simulink model "Follower_Agent"  (R2014b)
settings: Solver=ode3  SolverMode=SingleTasking  StartTime=0.0  StopTime=10.0  FixedStep=sampleTimes.main  RelTol=1e-3
model workspace (MAT data in the model file):
  vehicle = 0
undefined symbols (not defined in the file or in its folder): delays, sampleTimes
libraries: simulink x18
(part 1 of 2)
settings Model: ParameterArgumentNames=vehicle  Creator=uos  LastModifiedBy=uos

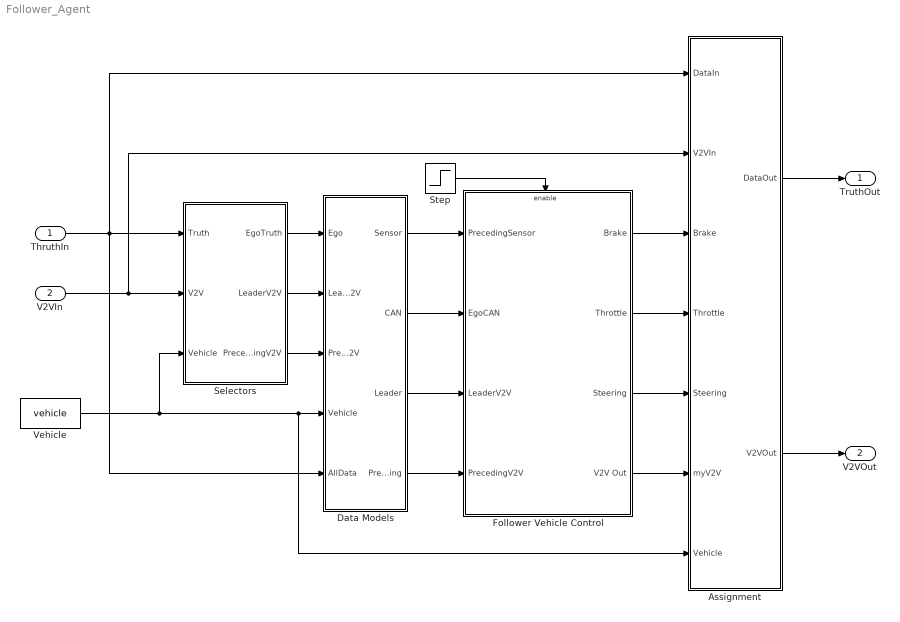
== system Follower_Agent ==
  ThruthIn : Inport  OutDataTypeStr=Bus: VehicleBus  PortDimensions=10  BusOutputAsStruct=on
  V2VIn : Inport  Port=2  OutDataTypeStr=Bus: V2VBus  PortDimensions=10  SampleTime=0  BusOutputAsStruct=on
  Assignment : Subsystem
  Data Models : Subsystem
  Follower Vehicle Control : Subsystem
  Selectors : Subsystem
  Step : Step  Time=vehicle*2  SampleTime=0
  Vehicle : Constant  Value=vehicle  OutDataTypeStr=int32
  TruthOut : Outport  OutDataTypeStr=Bus: VehicleBus  PortDimensions=10  BusOutputAsStruct=on
  V2VOut : Outport  Port=2  OutDataTypeStr=Bus: V2VBus  PortDimensions=10  BusOutputAsStruct=on
  wires:
  ThruthIn/1 -> Data Models/5(AllData), Assignment/1(DataIn), Selectors/1(Truth)
  Assignment/1(DataOut) -> TruthOut/1
  Vehicle/1 -> Data Models/4(Vehicle), Assignment/7(Vehicle), Selectors/3(Vehicle)
  Follower Vehicle Control/1(Brake) -> Assignment/3(Brake)
  Follower Vehicle Control/2(Throttle) -> Assignment/4(Throttle)
  Follower Vehicle Control/3(Steering) -> Assignment/5(Steering)
  V2VIn/1 -> Assignment/2(V2VIn), Selectors/2(V2V)
  Assignment/2(V2VOut) -> V2VOut/1
  Follower Vehicle Control/4(V2V Out) -> Assignment/6(myV2V)
  Selectors/1(EgoTruth) -> Data Models/1(Ego)
  Selectors/2(LeaderV2V) -> Data Models/2(LeaderV2V)
  Selectors/3(PrecedingV2V) -> Data Models/3(PrecedingV2V)
  Data Models/1(Sensor) -> Follower Vehicle Control/1(PrecedingSensor)
  Data Models/2(CAN) -> Follower Vehicle Control/2(EgoCAN)
  Data Models/3(Leader) -> Follower Vehicle Control/3(LeaderV2V)
  Data Models/4(Preceding) -> Follower Vehicle Control/4(PrecedingV2V)
  Step/1 -> Follower Vehicle Control/Enable

== system Follower_Agent/Assignment ==
  DataIn : Inport
  V2VIn : Inport  Port=2
  Brake : Inport  Port=3
  Throttle : Inport  Port=4
  Steering : Inport  Port=5
  myV2V : Inport  Port=6
  Vehicle : Inport  Port=7
  Clutch pedal value : Constant  Value=0
  Gear : Constant  Value=5  OutDataTypeStr=int32
  MATLAB Function : MATLAB Function  TreatAsAtomicUnit=on
  DataOut : Outport
  V2VOut : Outport  Port=2
  wires:
  Vehicle/1 -> MATLAB Function/9(vehicle)
  DataIn/1 -> MATLAB Function/1(dataIn)
  Brake/1 -> MATLAB Function/4(brake)
  MATLAB Function/1(dataOut) -> DataOut/1
  Throttle/1 -> MATLAB Function/5(throttle)
  Steering/1 -> MATLAB Function/8(steering)
  V2VIn/1 -> MATLAB Function/2(V2Vin)
  myV2V/1 -> MATLAB Function/3(myV2V)
  MATLAB Function/2(V2Vout) -> V2VOut/1
  Gear/1 -> MATLAB Function/6(gear)
  Clutch pedal value/1 -> MATLAB Function/7(clutch)

== system Follower_Agent/Data Models ==
  Ego : Inport
  LeaderV2V : Inport  Port=2
  PrecedingV2V : Inport  Port=3
  Vehicle : Inport  Port=4
  AllData : Inport  Port=5
  CAN Model : Subsystem
  Comms Model : Subsystem
  Sensor Model1 : Subsystem
  Sensor : Outport
  CAN : Outport  Port=2
  Leader : Outport  Port=3
  Preceding : Outport  Port=4
  wires:
  CAN Model/1(EgoCAN) -> CAN/1
  LeaderV2V/1 -> Comms Model/1(LeaderV2VIn)
  PrecedingV2V/1 -> Comms Model/2(PrecedingV2VIn)
  Comms Model/1(LeaderV2V) -> Leader/1
  Comms Model/2(PrecedingV2V) -> Preceding/1
  Vehicle/1 -> CAN Model/2(Vehicle), Sensor Model1/2(Vehicle)
  Ego/1 -> Sensor Model1/3(Ego), CAN Model/1(EgoData)
  AllData/1 -> Sensor Model1/1(AllData)
  Sensor Model1/1(Radar Data) -> Sensor/1

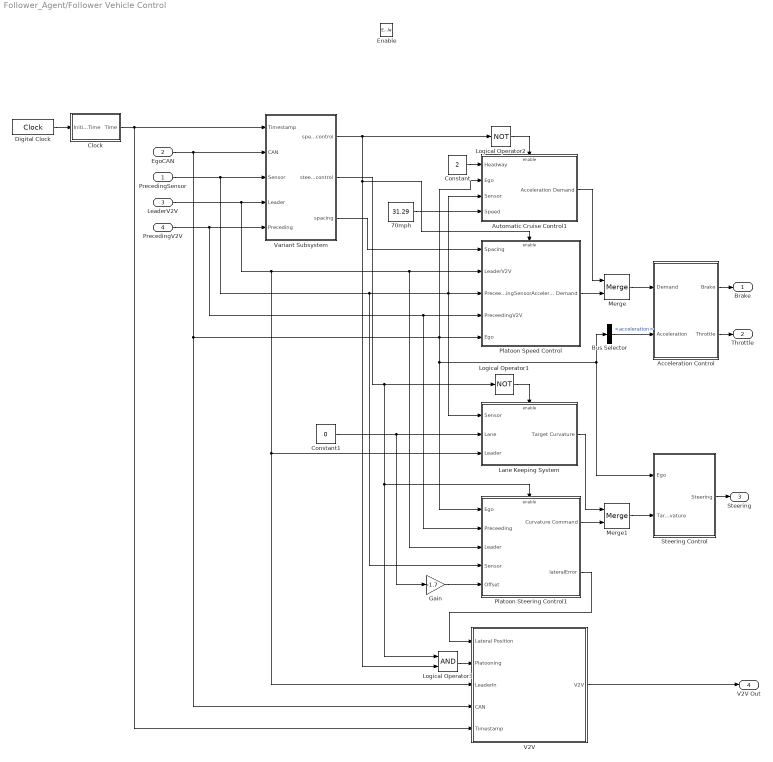
== system Follower_Agent/Follower Vehicle Control ==
  PrecedingSensor : Inport
  EgoCAN : Inport  Port=2
  LeaderV2V : Inport  Port=3
  PrecedingV2V : Inport  Port=4
  Enable : EnablePort
  70mph : Constant  Value=31.29
  Acceleration Control : Subsystem
  Automatic Cruise Control1 : Subsystem
  Bus Selector : BusSelector  OutputSignals=acceleration
  Clock : Subsystem
  Constant : Constant  Value=2
  Constant1 : Constant  Value=0
  Digital Clock : DigitalClock  SampleTime=sampleTimes.control
  Gain : Gain  Gain=-1.7
  Lane Keeping System : Subsystem
  Logical Operator1 : Logic  Operator=NOT  AllPortsSameDT=off  OutDataTypeStr=boolean
  Logical Operator2 : Logic  Operator=NOT  AllPortsSameDT=off  OutDataTypeStr=boolean
  Logical Operator3 : Logic  AllPortsSameDT=off  OutDataTypeStr=boolean
  Merge : Merge
  Merge1 : Merge
  Platoon Speed Control : Subsystem
  Platoon Steering Control1 : Subsystem
  Steering Control : Subsystem
  V2V : Subsystem
  Variant Subsystem : Subsystem  Variant=on  OverrideUsingVariant=Variant
  Brake : Outport
  Throttle : Outport  Port=2
  Steering : Outport  Port=3
  V2V Out : Outport  Port=4
  wires:
  Bus Selector/1 -> Acceleration Control/2(Acceleration)  "<acceleration>"
  Acceleration Control/1(Brake) -> Brake/1
  Acceleration Control/2(Throttle) -> Throttle/1
  Steering Control/1(Steering) -> Steering/1
  LeaderV2V/1 -> Variant Subsystem/4(Leader), Lane Keeping System/3(Leader), V2V/3(LeaderIn), Platoon Steering Control1/3(Leader), Platoon Speed Control/2(LeaderV2V)
  PrecedingSensor/1 -> Variant Subsystem/3(Sensor), Platoon Steering Control1/4(Sensor), Automatic Cruise Control1/3(Sensor), Lane Keeping System/1(Sensor), Platoon Speed Control/3(PreceedingSensor)
  Merge/1 -> Acceleration Control/1(Demand)
  Variant Subsystem/1(speed_control) -> Logical Operator3/2, Platoon Speed Control/Enable, Logical Operator2/1
  Merge1/1 -> Steering Control/2(Target Curvature)
  V2V/1(V2V) -> V2V Out/1
  PrecedingV2V/1 -> Variant Subsystem/5(Preceding), Platoon Steering Control1/2(Preceeding), Platoon Speed Control/4(PreceedingV2V)
  Digital Clock/1 -> Clock/1(Initial Time)
  Clock/1(Time) -> Variant Subsystem/1(Timestamp), V2V/5(Timestamp)
  Logical Operator2/1 -> Automatic Cruise Control1/Enable
  Constant/1 -> Automatic Cruise Control1/1(Headway)
  Variant Subsystem/3(spacing) -> Platoon Speed Control/1(Spacing)
  Automatic Cruise Control1/1(Acceleration Demand) -> Merge/1
  Platoon Speed Control/1(Acceleration Demand) -> Merge/2
  Logical Operator1/1 -> Lane Keeping System/Enable
  Variant Subsystem/2(steering_control) -> Logical Operator1/1, Platoon Steering Control1/Enable, Logical Operator3/1
  EgoCAN/1 -> Variant Subsystem/2(CAN), Automatic Cruise Control1/2(Ego), Platoon Steering Control1/1(Ego), Steering Control/1(Ego), Bus Selector/1, Platoon Speed Control/5(Ego), V2V/4(CAN)
  Lane Keeping System/1(Target Curvature) -> Merge1/1
  Platoon Steering Control1/1(Curvature Command) -> Merge1/2
  Platoon Steering Control1/2(lateralError) -> V2V/1(Lateral Position)
  Logical Operator3/1 -> V2V/2(Platooning)
  Constant1/1 -> Gain/1, Lane Keeping System/2(Lane)
  Gain/1 -> Platoon Steering Control1/5(Offset)
  70mph/1 -> Automatic Cruise Control1/4(Speed)

== system Follower_Agent/Selectors ==
  Truth : Inport
  V2V : Inport  Port=2
  Vehicle : Inport  Port=3
  MATLAB Function : MATLAB Function  TreatAsAtomicUnit=on
  EgoTruth : Outport
  LeaderV2V : Outport  Port=2
  PrecedingV2V : Outport  Port=3
  wires:
  Truth/1 -> MATLAB Function/1(data)
  Vehicle/1 -> MATLAB Function/3(vehicle)
  MATLAB Function/1(egoTruth) -> EgoTruth/1
  V2V/1 -> MATLAB Function/2(V2V)
  MATLAB Function/2(leaderV2V) -> LeaderV2V/1
  MATLAB Function/3(precedingV2V) -> PrecedingV2V/1

== system Follower_Agent/Data Models/CAN Model ==
  EgoData : Inport
  Vehicle : Inport  Port=2
  CAN Model : Subsystem
  EgoCAN : Outport
  wires:
  EgoData/1 -> CAN Model/1(Data)
  CAN Model/1(CAN) -> EgoCAN/1
  Vehicle/1 -> CAN Model/2(Vehicle)

== system Follower_Agent/Data Models/Comms Model ==
  LeaderV2VIn : Inport
  PrecedingV2VIn : Inport  Port=2
  Comms Delay : Subsystem
  Comms Delay1 : Subsystem
  Constant : Constant  Value=0
  Constant1 : Constant  Value=0
  LeaderV2V : Outport
  PrecedingV2V : Outport  Port=2
  wires:
  LeaderV2VIn/1 -> Comms Delay/1(Data)
  Comms Delay/1(V2V) -> LeaderV2V/1
  PrecedingV2VIn/1 -> Comms Delay1/1(Data)
  Comms Delay1/1(V2V) -> PrecedingV2V/1
  Constant/1 -> Comms Delay1/2(Delay)
  Constant1/1 -> Comms Delay/2(Delay)

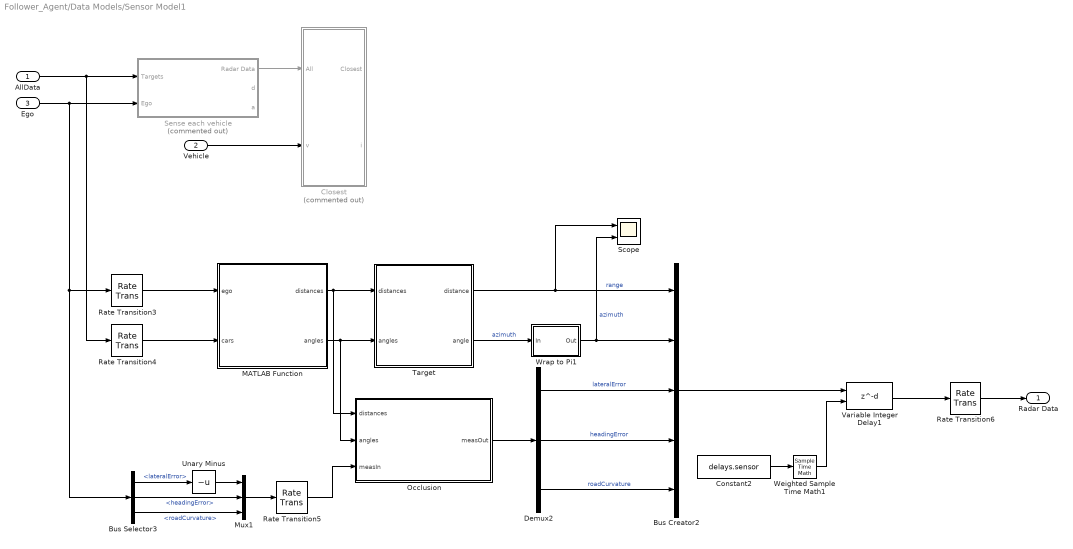
== system Follower_Agent/Data Models/Sensor Model1 ==
  AllData : Inport
  Vehicle : Inport  Port=2
  Ego : Inport  Port=3
  Bus Creator2 : BusCreator  Inputs=5  OutDataTypeStr=Bus: SensorData  NonVirtualBus=on
  Bus Selector3 : BusSelector  OutputSignals=data.lateralError,data.headingError,data.roadCurvature
  Closest : MATLAB Function  Commented=on  TreatAsAtomicUnit=on
  Constant2 : Constant  Value=delays.sensor
  Demux2 : Demux  Outputs=3
  MATLAB Function : MATLAB Function  TreatAsAtomicUnit=on
  Mux1 : Mux  Inputs=3
  Occlusion : MATLAB Function  TreatAsAtomicUnit=on
  Rate Transition3 : RateTransition  OutPortSampleTime=sampleTimes.main
  Rate Transition4 : RateTransition  OutPortSampleTime=sampleTimes.main
  Rate Transition5 : RateTransition  OutPortSampleTime=sampleTimes.main
  Rate Transition6 : RateTransition  OutPortSampleTime=sampleTimes.sensor
  Scope : Scope  NumInputPorts=2
      settings: TimeRange=23.7  YMin=0~-0.5  YMax=100~0
  Sense each vehicle : Subsystem  Commented=on  TreatAsAtomicUnit=on
  Target : MATLAB Function  TreatAsAtomicUnit=on
  Unary Minus : UnaryMinus
  Variable Integer Delay1 : Delay  DelayLengthSource=Input port
      settings: InputPortMap=u0,p1
  Weighted Sample Time Math1 : SampleTimeMath  TsampMathOp=/
  Wrap to Pi1 : Subsystem
  Radar Data : Outport
  wires:
  Vehicle/1 -> Closest/2(v)
  AllData/1 -> Rate Transition4/1, Sense each vehicle/1(Targets)
  Ego/1 -> Bus Selector3/1, Rate Transition3/1, Sense each vehicle/2(Ego)
  Sense each vehicle/1(Radar Data) -> Closest/1(All)
  Rate Transition3/1 -> MATLAB Function/1(ego)
  Rate Transition4/1 -> MATLAB Function/2(cars)
  MATLAB Function/1(distances) -> Occlusion/1(distances), Target/1(distances)
  MATLAB Function/2(angles) -> Occlusion/2(angles), Target/2(angles)
  Demux2/1 -> Bus Creator2/3  "lateralError"
  Demux2/2 -> Bus Creator2/4  "headingError"
  Demux2/3 -> Bus Creator2/5  "roadCurvature"
  Target/2(angle) -> Wrap to Pi1/1(In)  "azimuth"
  Target/1(distance) -> Scope/1, Bus Creator2/1  "range"
  Mux1/1 -> Rate Transition5/1
  Bus Selector3/1 -> Unary Minus/1  "<lateralError>"
  Bus Selector3/2 -> Mux1/2  "<headingError>"
  Bus Selector3/3 -> Mux1/3  "<roadCurvature>"
  Rate Transition5/1 -> Occlusion/3(measIn)
  Occlusion/1(measOut) -> Demux2/1
  Bus Creator2/1 -> Variable Integer Delay1/1
  Variable Integer Delay1/1 -> Rate Transition6/1
  Constant2/1 -> Weighted Sample Time Math1/1
  Weighted Sample Time Math1/1 -> Variable Integer Delay1/2
  Rate Transition6/1 -> Radar Data/1
  Wrap to Pi1/1(Out) -> Scope/2, Bus Creator2/2  "azimuth"
  Unary Minus/1 -> Mux1/1

== system Follower_Agent/Follower Vehicle Control/Acceleration Control ==
  Demand : Inport
  Acceleration : Inport  Port=2
  Brake Control : Subsystem
  Compare To Constant : simulink/Logic and Bit Operations/Compare To Constant  relop=>=  const=-0.1  OutDataTypeStr=boolean
  Logical Operator : Logic  Operator=NOT  AllPortsSameDT=off  OutDataTypeStr=boolean
  Sum1 : Sum  Inputs=+-|
  Throttle Control : Subsystem
  Brake : Outport
  Throttle : Outport  Port=2
  wires:
  Acceleration/1 -> Throttle Control/2(Acceleration), Sum1/2
  Demand/1 -> Throttle Control/1(Demand), Compare To Constant/1, Sum1/1
  Sum1/1 -> Brake Control/1(Error)
  Brake Control/1(Brake) -> Brake/1
  Throttle Control/1(Throttle) -> Throttle/1
  Compare To Constant/1 -> Throttle Control/Enable, Logical Operator/1
  Logical Operator/1 -> Brake Control/Enable

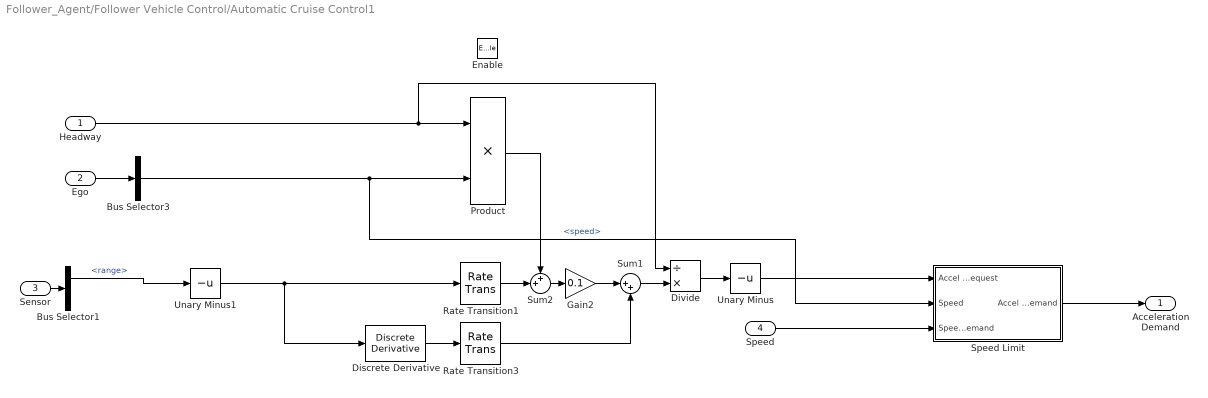
== system Follower_Agent/Follower Vehicle Control/Automatic Cruise Control1 ==
  Headway : Inport
  Ego : Inport  Port=2
  Sensor : Inport  Port=3
  Speed : Inport  Port=4
  Enable : EnablePort
  Bus Selector1 : BusSelector  OutputSignals=range,azimuth
  Bus Selector3 : BusSelector  OutputSignals=speed
  Discrete Derivative : simulink/Discrete/Discrete Derivative  gainval=1.0  ICPrevScaledInput=0.0  InputProcessing=Inherited  OutMin=[]  OutMax=[]  OutDataType=fixdt(1, 16)  OutScaling=2^-10  DoSatur=off
  Divide : Product  Inputs=/*
  Gain2 : Gain  Gain=0.1
  Product : Product
  Rate Transition1 : RateTransition  OutPortSampleTime=sampleTimes.control
  Rate Transition3 : RateTransition  OutPortSampleTime=sampleTimes.control
  Speed Limit : Subsystem
  Sum1 : Sum  Inputs=|++
  Sum2 : Sum  Inputs=++|
  Unary Minus : UnaryMinus
  Unary Minus1 : UnaryMinus
  Acceleration Demand : Outport
  wires:
  Ego/1 -> Bus Selector3/1
  Sensor/1 -> Bus Selector1/1
  Bus Selector3/1 -> Speed Limit/2(Speed), Product/2  "<speed>"
  Headway/1 -> Divide/1, Product/1
  Bus Selector1/1 -> Unary Minus1/1  "<range>"
  Product/1 -> Sum2/1
  Sum2/1 -> Gain2/1
  Gain2/1 -> Sum1/1
  Discrete Derivative/1 -> Rate Transition3/1
  Sum1/1 -> Divide/2
  Divide/1 -> Unary Minus/1
  Rate Transition3/1 -> Sum1/2
  Rate Transition1/1 -> Sum2/2
  Speed Limit/1(Accel Demand) -> Acceleration Demand/1
  Speed/1 -> Speed Limit/3(SpeedDemand)
  Unary Minus1/1 -> Discrete Derivative/1, Rate Transition1/1
  Unary Minus/1 -> Speed Limit/1(Accel Request)

== system Follower_Agent/Follower Vehicle Control/Clock ==
  Initial Time : Inport
  Constant : Constant
  Discrete-Time Integrator : DiscreteIntegrator  ExternalReset=either  InitialConditionSource=external  InitialConditionSetting=State (most efficient)  SampleTime=sampleTimes.control
  Time : Outport
  wires:
  Constant/1 -> Discrete-Time Integrator/1
  Initial Time/1 -> Discrete-Time Integrator/2, Discrete-Time Integrator/3
  Discrete-Time Integrator/1 -> Time/1

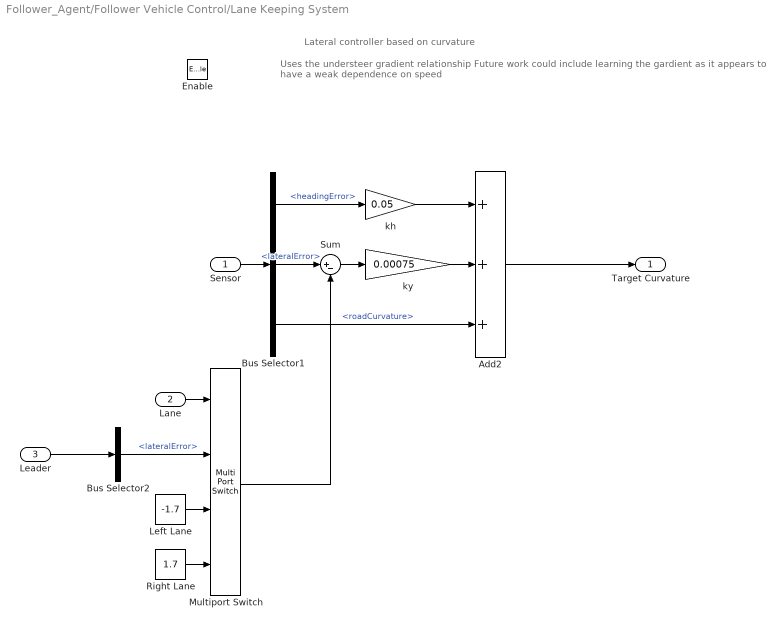
== system Follower_Agent/Follower Vehicle Control/Lane Keeping System ==
  note: Uses the understeer gradient relationship
      | Future work could include learning the gardient as it appears to have a weak dependence on speed
  note: Lateral controller based on curvature
  Sensor : Inport
  Lane : Inport  Port=2
  Leader : Inport  Port=3
  Enable : EnablePort
  Add2 : Sum  Inputs=+++
  Bus Selector1 : BusSelector  OutputSignals=headingError,lateralError,roadCurvature
  Bus Selector2 : BusSelector  OutputSignals=lateralError
  Left Lane : Constant  Value=-1.7
  Multiport Switch : MultiPortSwitch  DataPortOrder=Zero-based contiguous
  Right Lane : Constant  Value=1.7
  Sum : Sum  Inputs=|+-
  kh : Gain  Gain=0.05
  ky : Gain  Gain=0.00075
  Target Curvature : Outport
  wires:
  Sum/1 -> ky/1
  kh/1 -> Add2/1
  ky/1 -> Add2/2
  Add2/1 -> Target Curvature/1
  Sensor/1 -> Bus Selector1/1
  Bus Selector1/1 -> kh/1  "<headingError>"
  Bus Selector1/3 -> Add2/3  "<roadCurvature>"
  Bus Selector1/2 -> Sum/1  "<lateralError>"
  Multiport Switch/1 -> Sum/2
  Left Lane/1 -> Multiport Switch/3
  Right Lane/1 -> Multiport Switch/4
  Lane/1 -> Multiport Switch/1
  Leader/1 -> Bus Selector2/1
  Bus Selector2/1 -> Multiport Switch/2  "<lateralError>"

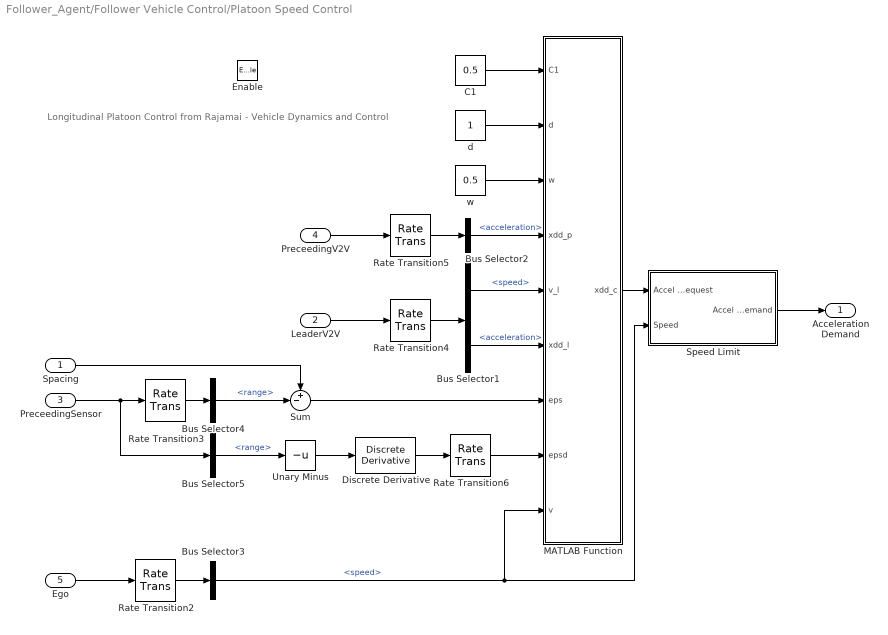
== system Follower_Agent/Follower Vehicle Control/Platoon Speed Control ==
  note: Longitudinal Platoon Control from Rajamai - Vehicle Dynamics and Control
  Spacing : Inport
  LeaderV2V : Inport  Port=2
  PreceedingSensor : Inport  Port=3
  PreceedingV2V : Inport  Port=4
  Ego : Inport  Port=5
  Enable : EnablePort
  Bus Selector1 : BusSelector  OutputSignals=speed,acceleration
  Bus Selector2 : BusSelector  OutputSignals=acceleration
  Bus Selector3 : BusSelector  OutputSignals=speed
  Bus Selector4 : BusSelector  OutputSignals=range
  Bus Selector5 : BusSelector  OutputSignals=range
  C1 : Constant  Value=0.5
  Discrete Derivative : simulink/Discrete/Discrete Derivative  gainval=1.0  ICPrevScaledInput=0.0  InputProcessing=Inherited  OutMin=[]  OutMax=[]  OutDataType=fixdt(1, 16)  OutScaling=2^-10  DoSatur=off
  MATLAB Function : MATLAB Function  TreatAsAtomicUnit=on
  Rate Transition2 : RateTransition  OutPortSampleTime=sampleTimes.control
  Rate Transition3 : RateTransition  OutPortSampleTime=sampleTimes.control
  Rate Transition4 : RateTransition  Deterministic=off  OutPortSampleTime=sampleTimes.control
  Rate Transition5 : RateTransition  Deterministic=off  OutPortSampleTime=sampleTimes.control
  Rate Transition6 : RateTransition  Deterministic=off  OutPortSampleTime=sampleTimes.control
  Speed Limit : Subsystem
  Sum : Sum  Inputs=+-|
  Unary Minus : UnaryMinus
  d : Constant
  w : Constant  Value=0.5
  Acceleration Demand : Outport
  wires:
  Ego/1 -> Rate Transition2/1
  Bus Selector3/1 -> Speed Limit/2(Speed), MATLAB Function/9(v)  "<speed>"
  PreceedingSensor/1 -> Bus Selector5/1, Rate Transition3/1
  Bus Selector4/1 -> Sum/2  "<range>"
  Discrete Derivative/1 -> Rate Transition6/1
  Speed Limit/1(Accel Demand) -> Acceleration Demand/1
  C1/1 -> MATLAB Function/1(C1)
  d/1 -> MATLAB Function/2(d)
  w/1 -> MATLAB Function/3(w)
  Spacing/1 -> Sum/1
  LeaderV2V/1 -> Rate Transition4/1
  Bus Selector1/2 -> MATLAB Function/6(xdd_l)  "<acceleration>"
  Bus Selector1/1 -> MATLAB Function/5(v_l)  "<speed>"
  PreceedingV2V/1 -> Rate Transition5/1
  Bus Selector2/1 -> MATLAB Function/4(xdd_p)  "<acceleration>"
  Rate Transition2/1 -> Bus Selector3/1
  Rate Transition3/1 -> Bus Selector4/1
  Rate Transition4/1 -> Bus Selector1/1
  Rate Transition5/1 -> Bus Selector2/1
  Bus Selector5/1 -> Unary Minus/1  "<range>"
  Rate Transition6/1 -> MATLAB Function/8(epsd)
  Sum/1 -> MATLAB Function/7(eps)
  Unary Minus/1 -> Discrete Derivative/1
  MATLAB Function/1(xdd_c) -> Speed Limit/1(Accel Request)

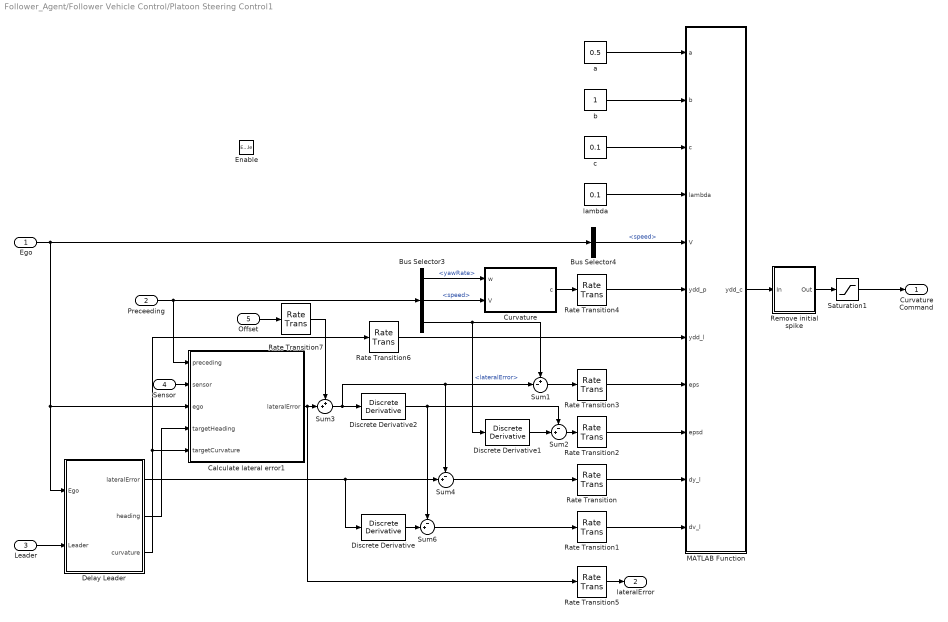
== system Follower_Agent/Follower Vehicle Control/Platoon Steering Control1 ==
  Ego : Inport
  Preceeding : Inport  Port=2
  Leader : Inport  Port=3
  Sensor : Inport  Port=4
  Offset : Inport  Port=5
  Enable : EnablePort
  Bus Selector3 : BusSelector  OutputSignals=yawRate,speed,lateralError
  Bus Selector4 : BusSelector  OutputSignals=speed
  Calculate lateral error1 : Subsystem
  Curvature : MATLAB Function  TreatAsAtomicUnit=on
  Delay Leader : Subsystem
  Discrete Derivative : simulink/Discrete/Discrete Derivative  gainval=1.0  ICPrevScaledInput=0.0  InputProcessing=Inherited  OutMin=[]  OutMax=[]  OutDataType=fixdt(1, 16)  OutScaling=2^-10  DoSatur=off
  Discrete Derivative1 : simulink/Discrete/Discrete Derivative  gainval=1.0  ICPrevScaledInput=0.0  InputProcessing=Inherited  OutMin=[]  OutMax=[]  OutDataType=fixdt(1, 16)  OutScaling=2^-10  DoSatur=off
  Discrete Derivative2 : simulink/Discrete/Discrete Derivative  gainval=1.0  ICPrevScaledInput=0.0  InputProcessing=Inherited  OutMin=[]  OutMax=[]  OutDataType=fixdt(1, 16)  OutScaling=2^-10  DoSatur=off
  MATLAB Function : MATLAB Function  TreatAsAtomicUnit=on
  Rate Transition : RateTransition  Integrity=off  Deterministic=off  OutPortSampleTime=sampleTimes.control
  Rate Transition{1..4,6} (5 alike) : RateTransition  OutPortSampleTime=sampleTimes.control
  Rate Transition5 : RateTransition  Integrity=off  Deterministic=off  OutPortSampleTime=sampleTimes.control
  Rate Transition7 : RateTransition  OutPortSampleTime=sampleTimes.v2v
  Remove initial spike : Subsystem
  Saturation1 : Saturate  UpperLimit=0.1  LowerLimit=-0.1
  Sum1 : Sum  Inputs=+-|
  Sum2 : Sum  Inputs=-+|
  Sum3 : Sum  Inputs=++|
  Sum4 : Sum  Inputs=-+|
  Sum6 : Sum  Inputs=-+|
  a : Constant  Value=0.5
  b : Constant
  c : Constant  Value=0.1
  lambda : Constant  Value=0.1
  Curvature Command : Outport
  lateralError : Outport  Port=2
  wires:
  Curvature/1(c) -> Rate Transition4/1
  Rate Transition/1 -> MATLAB Function/10(dy_l)
  Delay Leader/2(heading) -> Calculate lateral error1/4(targetHeading)
  Sum6/1 -> Rate Transition1/1
  Rate Transition1/1 -> MATLAB Function/11(dv_l)
  Leader/1 -> Delay Leader/2(Leader)
  Sum4/1 -> Rate Transition/1
  Preceeding/1 -> Calculate lateral error1/1(preceding), Bus Selector3/1
  Rate Transition2/1 -> MATLAB Function/9(epsd)
  Rate Transition4/1 -> MATLAB Function/6(ydd_p)
  c/1 -> MATLAB Function/3(c)
  b/1 -> MATLAB Function/2(b)
  a/1 -> MATLAB Function/1(a)
  Saturation1/1 -> Curvature Command/1
  Sensor/1 -> Calculate lateral error1/2(sensor)
  lambda/1 -> MATLAB Function/4(lambda)
  Bus Selector4/1 -> MATLAB Function/5(V)  "<speed>"
  Rate Transition5/1 -> lateralError/1
  Delay Leader/1(lateralError) -> Sum4/2, Discrete Derivative/1
  Ego/1 -> Bus Selector4/1, Calculate lateral error1/3(ego), Delay Leader/1(Ego)
  Rate Transition3/1 -> MATLAB Function/8(eps)
  Bus Selector3/3 -> Discrete Derivative1/1, Sum1/1  "<lateralError>"
  Bus Selector3/2 -> Curvature/2(V)  "<speed>"
  Bus Selector3/1 -> Curvature/1(w)  "<yawRate>"
  Delay Leader/3(curvature) -> Calculate lateral error1/5(targetCurvature), Rate Transition6/1
  Rate Transition6/1 -> MATLAB Function/7(ydd_l)
  Sum2/1 -> Rate Transition2/1
  Sum1/1 -> Rate Transition3/1
  Sum3/1 -> Sum4/1, Sum1/2, Discrete Derivative2/1
  MATLAB Function/1(ydd_c) -> Remove initial spike/1(In)
  Remove initial spike/1(Out) -> Saturation1/1
  Discrete Derivative1/1 -> Sum2/2
  Discrete Derivative/1 -> Sum6/2
  Discrete Derivative2/1 -> Sum6/1, Sum2/1
  Calculate lateral error1/1(lateralError) -> Rate Transition5/1, Sum3/2
  Offset/1 -> Rate Transition7/1
  Rate Transition7/1 -> Sum3/1

== system Follower_Agent/Follower Vehicle Control/Steering Control ==
  Ego : Inport
  Target Curvature : Inport  Port=2
  Bus Selector : BusSelector  OutputSignals=yawRate,speed
  Discrete-Time Integrator : DiscreteIntegrator  InitialCondition=0.0065  InitialConditionSetting=State (most efficient)  SampleTime=-1  LimitOutput=on  UpperSaturationLimit=0.5  LowerSaturationLimit=-0.5
  Divide : Product  Inputs=*/
  Gain : Gain  Gain=50
  Gain1 : Gain  Gain=5
  Saturation : Saturate  UpperLimit=inf  LowerLimit=1
  Saturation5 : Saturate
  Scope : Scope
  Sum : Sum  Inputs=|-+
  Sum1 : Sum  Inputs=++|
  Steering : Outport
  wires:
  Saturation5/1 -> Steering/1
  Sum1/1 -> Scope/1, Saturation5/1
  Target Curvature/1 -> Sum/2
  Ego/1 -> Bus Selector/1
  Bus Selector/2 -> Saturation/1  "<speed>"
  Bus Selector/1 -> Divide/1  "<yawRate>"
  Saturation/1 -> Divide/2
  Divide/1 -> Sum/1
  Gain/1 -> Discrete-Time Integrator/1
  Sum/1 -> Gain/1, Gain1/1
  Gain1/1 -> Sum1/2
  Discrete-Time Integrator/1 -> Sum1/1

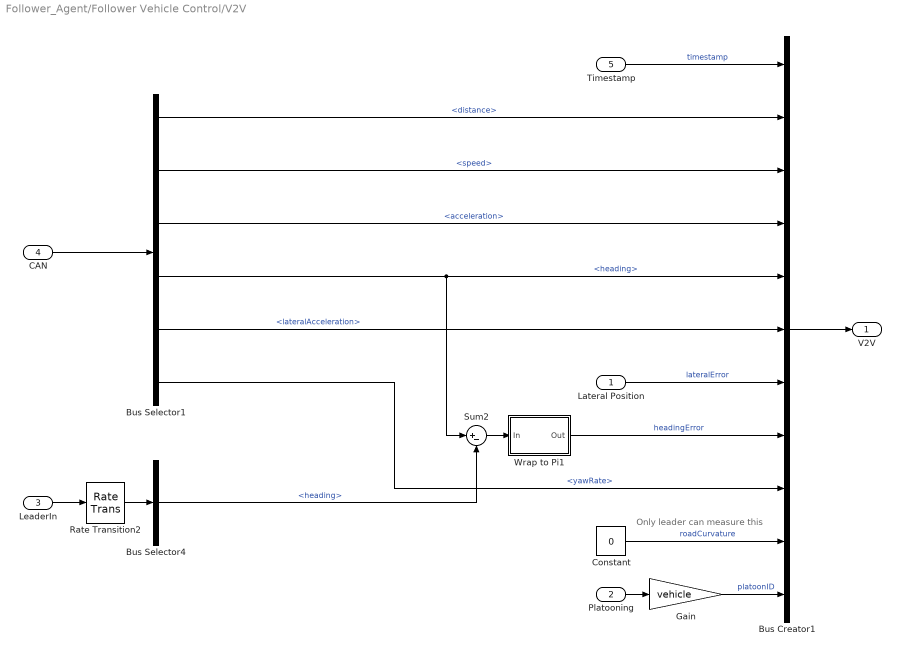
== system Follower_Agent/Follower Vehicle Control/V2V ==
  note: Only leader can measure this
  Lateral Position : Inport
  Platooning : Inport  Port=2
  LeaderIn : Inport  Port=3
  CAN : Inport  Port=4
  Timestamp : Inport  Port=5
  Bus Creator1 : BusCreator  Inputs=11  OutDataTypeStr=Bus: V2VBus  NonVirtualBus=on
  Bus Selector1 : BusSelector  OutputSignals=distance,speed,acceleration,heading,lateralAcceleration,yawRate
  Bus Selector4 : BusSelector  OutputSignals=heading
  Constant : Constant  Value=0
  Gain : Gain  Gain=vehicle  ParamDataTypeStr=int32  OutDataTypeStr=int32
  Rate Transition2 : RateTransition  OutPortSampleTime=sampleTimes.control
  Sum2 : Sum  Inputs=|+-
  Wrap to Pi1 : Subsystem
  V2V : Outport
  wires:
  CAN/1 -> Bus Selector1/1
  Bus Selector1/6 -> Bus Creator1/9  "<yawRate>"
  Constant/1 -> Bus Creator1/10  "roadCurvature"
  Bus Selector1/3 -> Bus Creator1/4  "<acceleration>"
  Bus Selector1/1 -> Bus Creator1/2  "<distance>"
  Bus Selector1/2 -> Bus Creator1/3  "<speed>"
  Bus Selector1/5 -> Bus Creator1/6  "<lateralAcceleration>"
  Bus Creator1/1 -> V2V/1
  Bus Selector1/4 -> Bus Creator1/5, Sum2/1  "<heading>"
  Sum2/1 -> Wrap to Pi1/1(In)
  LeaderIn/1 -> Rate Transition2/1
  Rate Transition2/1 -> Bus Selector4/1
  Bus Selector4/1 -> Sum2/2  "<heading>"
  Wrap to Pi1/1(Out) -> Bus Creator1/8  "headingError"
  Lateral Position/1 -> Bus Creator1/7  "lateralError"
  Platooning/1 -> Gain/1
  Timestamp/1 -> Bus Creator1/1  "timestamp"
  Gain/1 -> Bus Creator1/11  "platoonID"

== system Follower_Agent/Follower Vehicle Control/Variant Subsystem ==
  note: 1) Add Subsystem or Model blocks as valid variant choices.
      | 2) You cannot connect blocks at this level. At simulation, connectivity is automatically
      | determined, based on the active variant and port name matching.
  Timestamp : Inport
  CAN : Inport  Port=2
  Sensor : Inport  Port=3
  Leader : Inport  Port=4
  Preceding : Inport  Port=5
  Agent Control : Subsystem  VariantControl=Variant
  Non-Agent Control : Subsystem  VariantControl=Variant1
  speed_control : Outport
  steering_control : Outport  Port=2
  spacing : Outport  Port=3

== system Follower_Agent/Data Models/CAN Model/CAN Model ==
  Data : Inport
  Vehicle : Inport  Port=2
  Bus Creator : BusCreator  Inputs=7
  Bus Selector : BusSelector  OutputSignals=data.roadDistance,data.velocity,data.acceleration,data.angularVelocity,data.angle
  Gain : Gain
  Rate Transition1 : RateTransition  OutPortSampleTime=sampleTimes.main
  Selector : Selector  InputPortWidth=3
  Selector1 : Selector  InputPortWidth=3
  Selector2 : Selector  InputPortWidth=3  Indices=3
  Selector3 : Selector  InputPortWidth=3  Indices=2
  Selector4 : Selector  InputPortWidth=3  Indices=3
  CAN : Outport
  wires:
  Rate Transition1/1 -> CAN/1
  Bus Creator/1 -> Rate Transition1/1
  Selector1/1 -> Bus Creator/3  "acceleration"
  Bus Selector/3 -> Selector1/1, Selector3/1  "<acceleration>"
  Selector/1 -> Bus Creator/2  "speed"
  Bus Selector/2 -> Selector/1  "<velocity>"
  Data/1 -> Bus Selector/1
  Bus Selector/4 -> Selector2/1  "<angularVelocity>"
  Selector2/1 -> Bus Creator/5  "yawRate"
  Selector3/1 -> Bus Creator/4  "lateralAcceleration"
  Bus Selector/5 -> Selector4/1  "<angle>"
  Selector4/1 -> Bus Creator/6  "heading"
  Bus Selector/1 -> Gain/1  "<roadDistance>"
  Gain/1 -> Bus Creator/1  "distance"
  Vehicle/1 -> Bus Creator/7  "vehicle"

== system Follower_Agent/Data Models/Comms Model/Comms Delay ==
  Data : Inport
  Delay : Inport  Port=2
  Display : Display
  Rate Transition1 : RateTransition  OutPortSampleTime=sampleTimes.v2v
  Rate Transition2 : RateTransition  OutPortSampleTime=sampleTimes.main
  Variable Integer Delay : Delay  DelayLengthSource=Input port
      settings: InputPortMap=u0,p1
  Weighted Sample Time Math : SampleTimeMath  TsampMathOp=/
  V2V : Outport
  wires:
  Rate Transition1/1 -> V2V/1
  Data/1 -> Rate Transition2/1
  Rate Transition2/1 -> Variable Integer Delay/1
  Delay/1 -> Weighted Sample Time Math/1
  Weighted Sample Time Math/1 -> Display/1, Variable Integer Delay/2
  Variable Integer Delay/1 -> Rate Transition1/1

== system Follower_Agent/Data Models/Comms Model/Comms Delay1 ==
  Data : Inport
  Delay : Inport  Port=2
  Display : Display
  Rate Transition2 : RateTransition  OutPortSampleTime=sampleTimes.v2v
  Rate Transition3 : RateTransition  OutPortSampleTime=sampleTimes.main
  Variable Integer Delay : Delay  DelayLengthSource=Input port
      settings: InputPortMap=u0,p1
  Weighted Sample Time Math : SampleTimeMath  TsampMathOp=/
  V2V : Outport
  wires:
  Delay/1 -> Weighted Sample Time Math/1
  Rate Transition3/1 -> Variable Integer Delay/1
  Weighted Sample Time Math/1 -> Display/1, Variable Integer Delay/2
  Variable Integer Delay/1 -> Rate Transition2/1
  Data/1 -> Rate Transition3/1
  Rate Transition2/1 -> V2V/1

== system Follower_Agent/Data Models/Sensor Model1/Sense each vehicle ==
  Targets : Inport  Partition=on  PartitionDimension=1  PartitionWidth=1
  Ego : Inport  Port=2  Partition=off
  Bus Selector : BusSelector  OutputSignals=data.velocity
  For Each : ForEach  DisableCoverage=on  IndexMode=One-based
  Logical Operator : Logic  Operator=NOT  AllPortsSameDT=off  OutDataTypeStr=boolean
  Merge : Merge
  Non-zero : Subsystem
  Radar Model1 : Subsystem
  Radar Model2 : Subsystem
  Radar Data : Outport  OutDataTypeStr=Bus: SensorData  ConcatenationDimension=1
  d : Outport  Port=2  ConcatenationDimension=1
  a : Outport  Port=3  ConcatenationDimension=1
  wires:
  Targets/1 -> Bus Selector/1, Radar Model1/1(Target)
  Ego/1 -> Radar Model1/2(Ego)
  Radar Model1/1(Radar Data) -> Merge/1
  Radar Model2/1(Radar Data) -> Merge/2
  Merge/1 -> Radar Data/1
  Bus Selector/1 -> Non-zero/1(In1)  "<velocity>"
  Non-zero/1(Out1) -> Logical Operator/1, Radar Model1/Enable
  Logical Operator/1 -> Radar Model2/Enable
  Radar Model1/2(d) -> d/1
  Radar Model1/3(a) -> a/1

== system Follower_Agent/Data Models/Sensor Model1/Wrap to Pi1 ==
  In : Inport
  Bias : Bias  Bias=pi
  Bias1 : Bias  Bias=-pi
  Constant : Constant  Value=2*pi
  Math Function : Math  Operator=mod  SaturateOnIntegerOverflow=on
  Out : Outport
  wires:
  In/1 -> Bias/1
  Bias/1 -> Math Function/1
  Math Function/1 -> Bias1/1
  Bias1/1 -> Out/1
  Constant/1 -> Math Function/2

== system Follower_Agent/Follower Vehicle Control/Acceleration Control/Brake Control ==
  Error : Inport
  Enable : EnablePort  StatesWhenEnabling=reset
  Discrete-Time Integrator : DiscreteIntegrator  InitialConditionSetting=State (most efficient)  SampleTime=-1  LimitOutput=on  UpperSaturationLimit=1  LowerSaturationLimit=-1
  Gain2 : Gain  Gain=0.005
  Gain3 : Gain
  Saturation1 : Saturate  UpperLimit=1  LowerLimit=0
  Sum2 : Sum  Inputs=++|
  Unary Minus : UnaryMinus
  Brake : Outport  OutputWhenDisabled=reset  InitialOutput=0
  wires:
  Saturation1/1 -> Brake/1
  Sum2/1 -> Saturation1/1
  Error/1 -> Unary Minus/1
  Gain2/1 -> Sum2/2
  Discrete-Time Integrator/1 -> Sum2/1
  Gain3/1 -> Discrete-Time Integrator/1
  Unary Minus/1 -> Gain2/1, Gain3/1

== system Follower_Agent/Follower Vehicle Control/Acceleration Control/Throttle Control ==
  Demand : Inport
  Acceleration : Inport  Port=2
  Enable : EnablePort  StatesWhenEnabling=reset
  Discrete-Time Integrator : DiscreteIntegrator  InitialConditionSetting=State (most efficient)  SampleTime=-1  LimitOutput=on  UpperSaturationLimit=1  LowerSaturationLimit=-1
  Gain : Gain  Gain=1.5
  Gain1 : Gain  Gain=10
  Sum : Sum  Inputs=++|
  Sum1 : Sum  Inputs=+-|
  Throttle : Outport  OutputWhenDisabled=reset  InitialOutput=0
  wires:
  Gain/1 -> Sum/1
  Discrete-Time Integrator/1 -> Sum/2
  Gain1/1 -> Discrete-Time Integrator/1
  Sum/1 -> Throttle/1
  Demand/1 -> Sum1/1, Gain/1
  Acceleration/1 -> Sum1/2
  Sum1/1 -> Gain1/1

== system Follower_Agent/Follower Vehicle Control/Automatic Cruise Control1/Speed Limit ==
  Accel Request : Inport
  Speed : Inport  Port=2
  SpeedDemand : Inport  Port=3
  Compare To Zero : simulink/Logic and Bit Operations/Compare To Zero  relop=<  OutDataTypeStr=boolean
  Constant3 : Constant  Value=0
  Logical Operator : Logic  Operator=OR  AllPortsSameDT=off  OutDataTypeStr=boolean
  Relational Operator : RelationalOperator  Operator=<=  OutDataTypeStr=boolean
  Switch : Switch  Criteria=u2 > Threshold
  Accel Demand : Outport
  wires:
  Speed/1 -> Relational Operator/1
  Compare To Zero/1 -> Logical Operator/1
  Logical Operator/1 -> Switch/2
  Relational Operator/1 -> Logical Operator/2
  Constant3/1 -> Switch/3
  Accel Request/1 -> Compare To Zero/1, Switch/1
  Switch/1 -> Accel Demand/1
  SpeedDemand/1 -> Relational Operator/2

== system Follower_Agent/Follower Vehicle Control/Platoon Speed Control/Speed Limit ==
  Accel Request : Inport
  Speed : Inport  Port=2
  70mph : simulink/Logic and Bit Operations/Compare To Constant  relop=<  const=31.3  OutDataTypeStr=boolean
  Compare To Zero : simulink/Logic and Bit Operations/Compare To Zero  relop=<  OutDataTypeStr=boolean
  Constant3 : Constant  Value=0
  Logical Operator : Logic  Operator=OR  AllPortsSameDT=off  OutDataTypeStr=boolean
  Switch : Switch  Criteria=u2 > Threshold
  Accel Demand : Outport
  wires:
  Speed/1 -> 70mph/1
  Compare To Zero/1 -> Logical Operator/1
  Logical Operator/1 -> Switch/2
  70mph/1 -> Logical Operator/2
  Constant3/1 -> Switch/3
  Accel Request/1 -> Compare To Zero/1, Switch/1
  Switch/1 -> Accel Demand/1

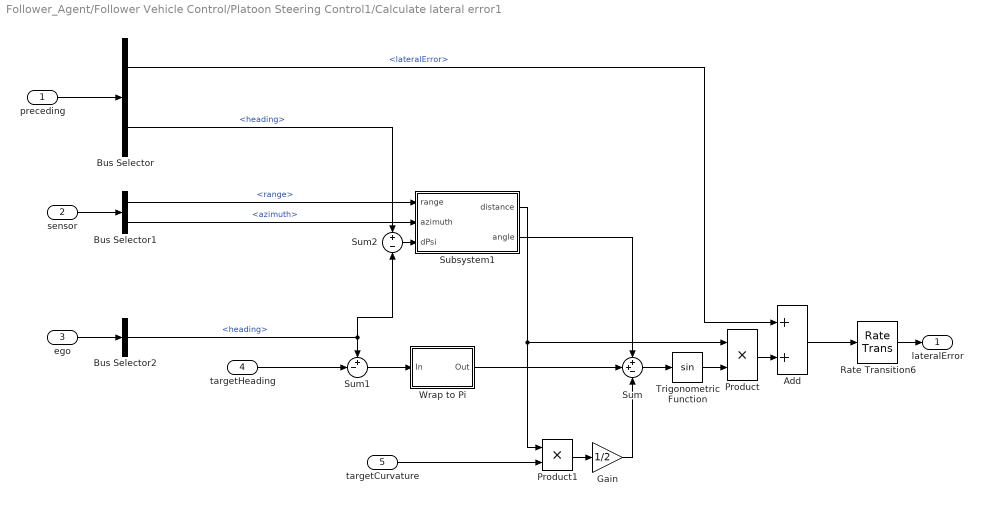
== system Follower_Agent/Follower Vehicle Control/Platoon Steering Control1/Calculate lateral error1 ==
  preceding : Inport
  sensor : Inport  Port=2
  ego : Inport  Port=3
  targetHeading : Inport  Port=4
  targetCurvature : Inport  Port=5
  Add : Sum
  Bus Selector : BusSelector  OutputSignals=lateralError,heading
  Bus Selector1 : BusSelector  OutputSignals=range,azimuth
  Bus Selector2 : BusSelector  OutputSignals=heading
  Gain : Gain  Gain=1/2
  Product : Product
  Product1 : Product
  Rate Transition6 : RateTransition  Integrity=off  OutPortSampleTime=sampleTimes.v2v
  Subsystem1 : Subsystem
  Sum : Sum  Inputs=++-
  Sum1 : Sum  Inputs=+-|
  Sum2 : Sum  Inputs=+|-
  Trigonometric Function : Trigonometry
  Wrap to Pi : Subsystem
  lateralError : Outport
  wires:
  Sum1/1 -> Wrap to Pi/1(In)
  Gain/1 -> Sum/3
  Product1/1 -> Gain/1
  Product/1 -> Add/2
  Bus Selector2/1 -> Sum2/2, Sum1/1  "<heading>"
  Sum/1 -> Trigonometric Function/1
  ego/1 -> Bus Selector2/1
  Add/1 -> Rate Transition6/1
  Sum2/1 -> Subsystem1/3(dPsi)
  Bus Selector/2 -> Sum2/1  "<heading>"
  Subsystem1/1(distance) -> Product1/1, Product/1
  Trigonometric Function/1 -> Product/2
  Wrap to Pi/1(Out) -> Sum/2
  Subsystem1/2(angle) -> Sum/1
  Bus Selector1/1 -> Subsystem1/1(range)  "<range>"
  Bus Selector1/2 -> Subsystem1/2(azimuth)  "<azimuth>"
  sensor/1 -> Bus Selector1/1
  Rate Transition6/1 -> lateralError/1
  targetHeading/1 -> Sum1/2
  targetCurvature/1 -> Product1/2
  Bus Selector/1 -> Add/1  "<lateralError>"
  preceding/1 -> Bus Selector/1

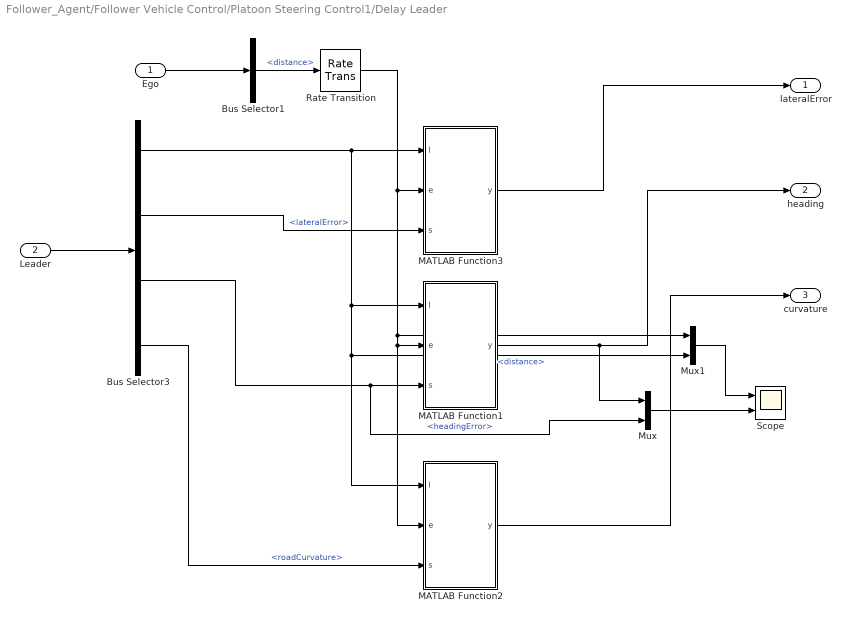
== system Follower_Agent/Follower Vehicle Control/Platoon Steering Control1/Delay Leader ==
  Ego : Inport
  Leader : Inport  Port=2
  Bus Selector1 : BusSelector  OutputSignals=distance
  Bus Selector3 : BusSelector  OutputSignals=distance,lateralError,headingError,roadCurvature
  MATLAB Function1 : MATLAB Function  TreatAsAtomicUnit=on
  MATLAB Function2 : MATLAB Function  TreatAsAtomicUnit=on
  MATLAB Function3 : MATLAB Function  TreatAsAtomicUnit=on
  Mux : Mux  Inputs=2
  Mux1 : Mux  Inputs=2
  Rate Transition : RateTransition  OutPortSampleTime=sampleTimes.v2v
  Scope : Scope  NumInputPorts=2
      settings: TimeRange=50.40000000000001  YMin=0~-5  YMax=12000~5  SaveName=ScopeData10
  lateralError : Outport
  heading : Outport  Port=2
  curvature : Outport  Port=3
  wires:
  MATLAB Function2/1(y) -> curvature/1
  Bus Selector3/4 -> MATLAB Function2/3(s)  "<roadCurvature>"
  MATLAB Function1/1(y) -> heading/1, Mux/1
  Bus Selector3/3 -> MATLAB Function1/3(s), Mux/2  "<headingError>"
  Mux1/1 -> Scope/1
  MATLAB Function3/1(y) -> lateralError/1
  Bus Selector3/2 -> MATLAB Function3/3(s)  "<lateralError>"
  Rate Transition/1 -> Mux1/1, MATLAB Function1/2(e), MATLAB Function2/2(e), MATLAB Function3/2(e)
  Bus Selector3/1 -> Mux1/2, MATLAB Function2/1(l), MATLAB Function1/1(l), MATLAB Function3/1(l)  "<distance>"
  Mux/1 -> Scope/2
  Bus Selector1/1 -> Rate Transition/1  "<distance>"
  Ego/1 -> Bus Selector1/1
  Leader/1 -> Bus Selector3/1

== system Follower_Agent/Follower Vehicle Control/Platoon Steering Control1/Remove initial spike ==
  In : Inport
  Compare To Constant : simulink/Logic and Bit Operations/Compare To Constant  relop=>  const=0.5  OutDataTypeStr=boolean
  Constant3 : Constant  Value=0
  Counter Free-Running : simulink/Sources/Counter Free-Running  NumBits=16  tsamp=-1
  Switch : Switch  Criteria=u2 > Threshold
  Weighted Sample Time Math : SampleTimeMath  TsampMathOp=*  weightValue=int32(1)  TsampMathImp=Offline Scaling Adjustment
  Out : Outport
  wires:
  In/1 -> Switch/1
  Switch/1 -> Out/1
  Counter Free-Running/1 -> Weighted Sample Time Math/1
  Weighted Sample Time Math/1 -> Compare To Constant/1
  Compare To Constant/1 -> Switch/2
  Constant3/1 -> Switch/3

== system Follower_Agent/Follower Vehicle Control/V2V/Wrap to Pi1 ==
  In : Inport
  Bias : Bias  Bias=pi
  Bias1 : Bias  Bias=-pi
  Constant : Constant  Value=2*pi
  Math Function : Math  Operator=mod  SaturateOnIntegerOverflow=on
  Out : Outport
  wires:
  Constant/1 -> Math Function/2
  Bias1/1 -> Out/1
  Math Function/1 -> Bias1/1
  Bias/1 -> Math Function/1
  In/1 -> Bias/1

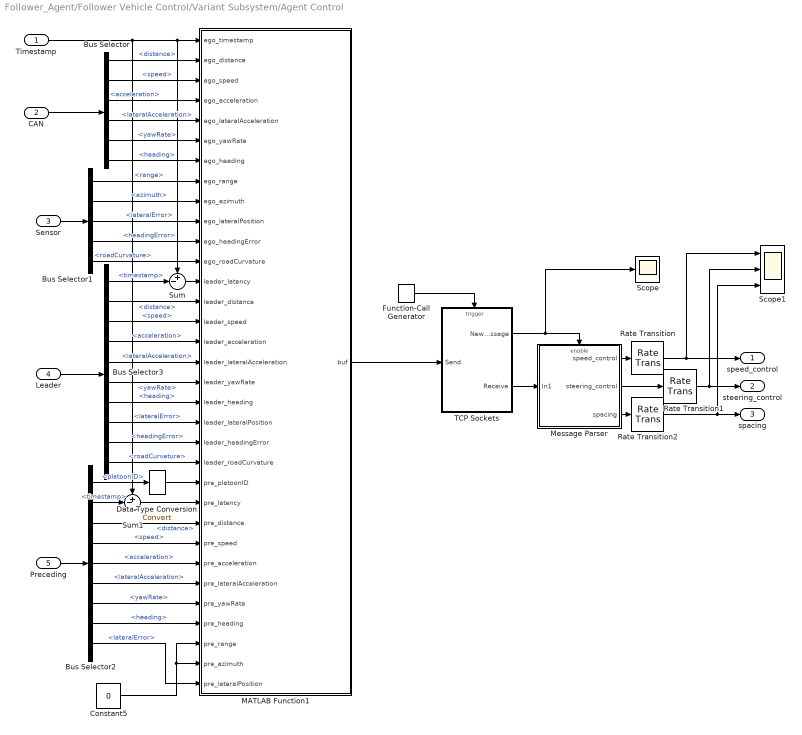
== system Follower_Agent/Follower Vehicle Control/Variant Subsystem/Agent Control ==
  Timestamp : Inport
  CAN : Inport  Port=2
  Sensor : Inport  Port=3
  Leader : Inport  Port=4
  Preceding : Inport  Port=5
  Bus Selector : BusSelector  OutputSignals=distance,speed,acceleration,lateralAcceleration,yawRate,heading
  Bus Selector1 : BusSelector  OutputSignals=range,azimuth,lateralError,headingError,roadCurvature
  Bus Selector2 : BusSelector  OutputSignals=platoonID,timestamp,distance,speed,acceleration,lateralAcceleration,yawRate,heading,lateralError
  Bus Selector3 : BusSelector  OutputSignals=timestamp,distance,speed,acceleration,lateralAcceleration,yawRate,heading,lateralError,headingError,roadCurvature
  Constant5 : Constant  Value=0
  Data Type Conversion : DataTypeConversion
  Function-Call Generator : simulink/Ports & Subsystems/Function-Call Generator  sample_time=1  numberOfIterations=1
  MATLAB Function1 : MATLAB Function  TreatAsAtomicUnit=on
  Message Parser : Subsystem  TreatAsAtomicUnit=on
  Rate Transition : RateTransition
  Rate Transition1 : RateTransition
  Rate Transition2 : RateTransition
  Scope : Scope
      settings: SaveName=ScopeData2
  Scope1 : Scope  NumInputPorts=3
      settings: YMin=-5~-5~-5  YMax=5~5~5  SaveName=ScopeData3
  Sum : Sum  Inputs=+-|
  Sum1 : Sum  Inputs=+-|
  TCP Sockets : Subsystem  TreatAsAtomicUnit=on
  speed_control : Outport
  steering_control : Outport  Port=2
  spacing : Outport  Port=3
  wires:
  Bus Selector3/6 -> MATLAB Function1/18(leader_yawRate)  "<yawRate>"
  Bus Selector3/7 -> MATLAB Function1/19(leader_heading)  "<heading>"
  Bus Selector3/8 -> MATLAB Function1/20(leader_lateralPosition)  "<lateralError>"
  Bus Selector3/9 -> MATLAB Function1/21(leader_headingError)  "<headingError>"
  Bus Selector2/3 -> MATLAB Function1/25(pre_distance)  "<distance>"
  Bus Selector2/7 -> MATLAB Function1/29(pre_yawRate)  "<yawRate>"
  Bus Selector2/4 -> MATLAB Function1/26(pre_speed)  "<speed>"
  Bus Selector2/5 -> MATLAB Function1/27(pre_acceleration)  "<acceleration>"
  Bus Selector2/9 -> MATLAB Function1/33(pre_lateralPosition)  "<lateralError>"
  Bus Selector2/8 -> MATLAB Function1/30(pre_heading)  "<heading>"
  Bus Selector2/6 -> MATLAB Function1/28(pre_lateralAcceleration)  "<lateralAcceleration>"
  Constant5/1 -> MATLAB Function1/32(pre_azimuth), MATLAB Function1/31(pre_range)
  Timestamp/1 -> Sum1/1, Sum/1, MATLAB Function1/1(ego_timestamp)
  TCP Sockets/2(Receive) -> Message Parser/1(In1)
  Function-Call Generator/1 -> TCP Sockets/Trigger
  Bus Selector2/1 -> Data Type Conversion/1  "<platoonID>"
  Data Type Conversion/1 -> MATLAB Function1/23(pre_platoonID)
  Message Parser/1(speed_control) -> Rate Transition/1
  TCP Sockets/1(NewMessage) -> Scope/1, Message Parser/Enable
  Message Parser/2(steering_control) -> Rate Transition1/1
  Message Parser/3(spacing) -> Rate Transition2/1
  Rate Transition/1 -> Scope1/1, speed_control/1
  Rate Transition1/1 -> Scope1/2, steering_control/1
  Rate Transition2/1 -> Scope1/3, spacing/1
  CAN/1 -> Bus Selector/1
  Sensor/1 -> Bus Selector1/1
  Preceding/1 -> Bus Selector2/1
  Leader/1 -> Bus Selector3/1
  MATLAB Function1/1(buf) -> TCP Sockets/1(Send)
  Bus Selector/1 -> MATLAB Function1/2(ego_distance)  "<distance>"
  Bus Selector/2 -> MATLAB Function1/3(ego_speed)  "<speed>"
  Bus Selector/3 -> MATLAB Function1/4(ego_acceleration)  "<acceleration>"
  Bus Selector/4 -> MATLAB Function1/5(ego_lateralAcceleration)  "<lateralAcceleration>"
  Bus Selector/5 -> MATLAB Function1/6(ego_yawRate)  "<yawRate>"
  Bus Selector/6 -> MATLAB Function1/7(ego_heading)  "<heading>"
  Bus Selector1/4 -> MATLAB Function1/11(ego_headingError)  "<headingError>"
  Bus Selector1/5 -> MATLAB Function1/12(ego_roadCurvature)  "<roadCurvature>"
  Bus Selector1/3 -> MATLAB Function1/10(ego_lateralPosition)  "<lateralError>"
  Bus Selector1/2 -> MATLAB Function1/9(ego_azimuth)  "<azimuth>"
  Bus Selector1/1 -> MATLAB Function1/8(ego_range)  "<range>"
  Bus Selector3/2 -> MATLAB Function1/14(leader_distance)  "<distance>"
  Bus Selector3/3 -> MATLAB Function1/15(leader_speed)  "<speed>"
  Bus Selector3/4 -> MATLAB Function1/16(leader_acceleration)  "<acceleration>"
  Bus Selector3/10 -> MATLAB Function1/22(leader_roadCurvature)  "<roadCurvature>"
  Bus Selector3/5 -> MATLAB Function1/17(leader_lateralAcceleration)  "<lateralAcceleration>"
  Sum/1 -> MATLAB Function1/13(leader_latency)
  Bus Selector3/1 -> Sum/2  "<timestamp>"
  Sum1/1 -> MATLAB Function1/24(pre_latency)
  Bus Selector2/2 -> Sum1/2  "<timestamp>"

== system Follower_Agent/Follower Vehicle Control/Variant Subsystem/Non-Agent Control ==
  Timestamp : Inport
  CAN : Inport  Port=2
  Sensor : Inport  Port=3
  Leader : Inport  Port=4
  Preceding : Inport  Port=5
  Bus Selector1 : BusSelector  OutputSignals=speed
  Bus Selector2 : BusSelector  OutputSignals=range,azimuth
  Bus Selector3 : BusSelector  OutputSignals=platoonID
  Enable Platooning : Stateflow chart  TreatAsAtomicUnit=on
  speed_control : Outport
  steering_control : Outport  Port=2
  spacing : Outport  Port=3
  wires:
  Bus Selector1/1 -> Enable Platooning/1(speed)  "<speed>"
  Preceding/1 -> Bus Selector3/1
  CAN/1 -> Bus Selector1/1
  Bus Selector2/1 -> Enable Platooning/2(distance)  "<range>"
  Bus Selector3/1 -> Enable Platooning/4(prePlatooning)  "<platoonID>"
  Sensor/1 -> Bus Selector2/1
  Bus Selector2/2 -> Enable Platooning/3(azimuth)  "<azimuth>"
  Enable Platooning/1(speedControl) -> speed_control/1
  Enable Platooning/2(steeringControl) -> steering_control/1
  Enable Platooning/4(spacing) -> spacing/1

== system Follower_Agent/Data Models/Sensor Model1/Sense each vehicle/Non-zero ==
  In1 : Inport
  Bias : Bias  Bias=-eps
  Compare To Zero : simulink/Logic and Bit Operations/Compare To Zero  relop=>  OutDataTypeStr=boolean
  Logical Operator : Logic  Inputs=1  AllPortsSameDT=off  OutDataTypeStr=boolean
  Norm : Subsystem
  Out1 : Outport
  wires:
  Compare To Zero/1 -> Logical Operator/1
  Logical Operator/1 -> Out1/1
  In1/1 -> Norm/1(In1)
  Norm/1(Out1) -> Bias/1
  Bias/1 -> Compare To Zero/1

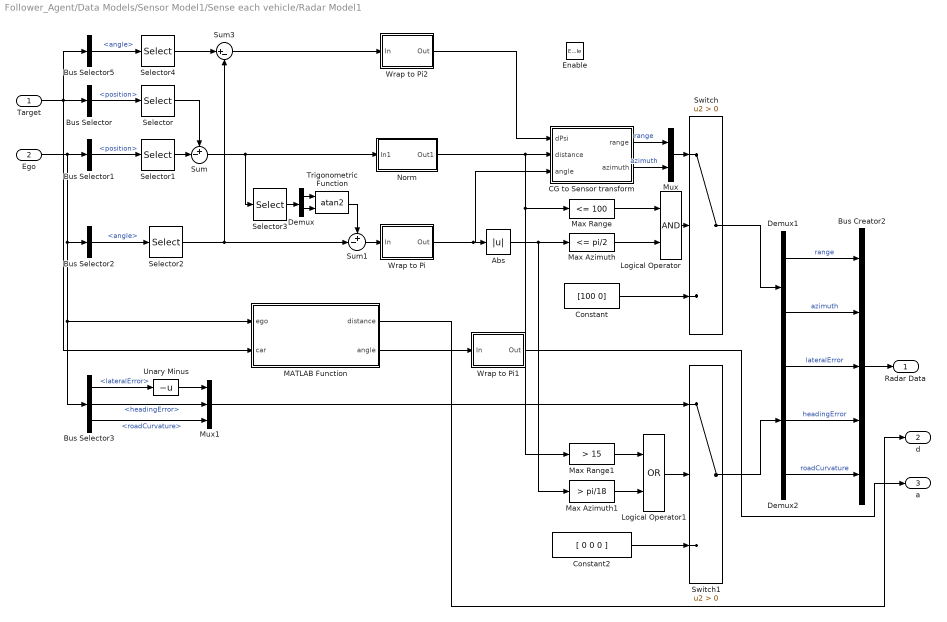
== system Follower_Agent/Data Models/Sensor Model1/Sense each vehicle/Radar Model1 ==
  Target : Inport
  Ego : Inport  Port=2
  Enable : EnablePort
  Abs : Abs
  Bus Creator2 : BusCreator  Inputs=5  OutDataTypeStr=Bus: SensorData  NonVirtualBus=on
  Bus Selector : BusSelector  OutputSignals=data.position
  Bus Selector1 : BusSelector  OutputSignals=data.position
  Bus Selector2 : BusSelector  OutputSignals=data.angle
  Bus Selector3 : BusSelector  OutputSignals=data.lateralError,data.headingError,data.roadCurvature
  Bus Selector5 : BusSelector  OutputSignals=data.angle
  CG to Sensor transform : Subsystem
  Constant : Constant  Value=[100 0]
  Constant2 : Constant  Value=[ 0 0 0 ]
  Demux : Demux  Outputs=2
  Demux1 : Demux  Outputs=2
  Demux2 : Demux  Outputs=3
  Logical Operator : Logic  AllPortsSameDT=off  OutDataTypeStr=boolean
  Logical Operator1 : Logic  Operator=OR  AllPortsSameDT=off  OutDataTypeStr=boolean
  MATLAB Function : MATLAB Function  TreatAsAtomicUnit=on
  Max Azimuth : simulink/Logic and Bit Operations/Compare To Constant  relop=<=  const=pi/2  OutDataTypeStr=boolean
  Max Azimuth1 : simulink/Logic and Bit Operations/Compare To Constant  relop=>  const=pi/18  OutDataTypeStr=boolean
  Max Range : simulink/Logic and Bit Operations/Compare To Constant  relop=<=  const=100  OutDataTypeStr=boolean
  Max Range1 : simulink/Logic and Bit Operations/Compare To Constant  relop=>  const=15  OutDataTypeStr=boolean
  Mux : Mux  Inputs=2
  Mux1 : Mux  Inputs=3
  Norm : Subsystem
  Selector : Selector  InputPortWidth=3  Indices=[1 2]
  Selector1 : Selector  InputPortWidth=3  Indices=[1 2]
  Selector2 : Selector  InputPortWidth=3  Indices=3
  Selector3 : Selector  InputPortWidth=2  Indices=[2 1]
  Selector4 : Selector  InputPortWidth=3  Indices=3
  Sum : Sum  Inputs=+-|
  Sum1 : Sum  Inputs=+-|
  Sum3 : Sum  Inputs=|+-
  Switch : Switch  Criteria=u2 > Threshold
  Switch1 : Switch  Criteria=u2 > Threshold
  Trigonometric Function : Trigonometry  Operator=atan2
  Unary Minus : UnaryMinus
  Wrap to Pi : Subsystem
  Wrap to Pi1 : Subsystem
  Wrap to Pi2 : Subsystem
  Radar Data : Outport
  d : Outport  Port=2
  a : Outport  Port=3
  wires:
  Selector1/1 -> Sum/2
  Selector/1 -> Sum/1
  Bus Selector/1 -> Selector/1  "<position>"
  Bus Selector1/1 -> Selector1/1  "<position>"
  Bus Selector2/1 -> Selector2/1  "<angle>"
  Sum/1 -> Selector3/1, Norm/1(In1)
  Selector2/1 -> Sum1/2, Sum3/2
  Trigonometric Function/1 -> Sum1/1
  Sum1/1 -> Wrap to Pi/1(In)
  Constant/1 -> Switch/3
  Logical Operator/1 -> Switch/2
  Max Range/1 -> Logical Operator/1
  Max Azimuth/1 -> Logical Operator/2
  Wrap to Pi/1(Out) -> CG to Sensor transform/3(angle), Abs/1
  Bus Creator2/1 -> Radar Data/1
  Switch/1 -> Demux1/1
  Ego/1 -> Bus Selector3/1, MATLAB Function/1(ego), Bus Selector2/1, Bus Selector1/1
  Mux1/1 -> Switch1/1
  Bus Selector3/1 -> Unary Minus/1  "<lateralError>"
  Bus Selector3/2 -> Mux1/2  "<headingError>"
  Max Range1/1 -> Logical Operator1/1
  Constant2/1 -> Switch1/3
  Switch1/1 -> Demux2/1
  Demux2/1 -> Bus Creator2/3  "lateralError"
  Demux2/2 -> Bus Creator2/4  "headingError"
  Bus Selector3/3 -> Mux1/3  "<roadCurvature>"
  Demux2/3 -> Bus Creator2/5  "roadCurvature"
  Unary Minus/1 -> Mux1/1
  Bus Selector5/1 -> Selector4/1  "<angle>"
  Target/1 -> MATLAB Function/2(car), Bus Selector5/1, Bus Selector/1
  Selector4/1 -> Sum3/1
  Sum3/1 -> Wrap to Pi2/1(In)
  Demux1/1 -> Bus Creator2/1  "range"
  Demux1/2 -> Bus Creator2/2  "azimuth"
  Logical Operator1/1 -> Switch1/2
  Max Azimuth1/1 -> Logical Operator1/2
  Abs/1 -> Max Azimuth1/1, Max Azimuth/1
  Mux/1 -> Switch/1
  CG to Sensor transform/1(range) -> Mux/1  "range"
  CG to Sensor transform/2(azimuth) -> Mux/2  "azimuth"
  Wrap to Pi2/1(Out) -> CG to Sensor transform/1(dPsi)
  Norm/1(Out1) -> Max Range1/1, Max Range/1, CG to Sensor transform/2(distance)
  Demux/2 -> Trigonometric Function/2
  Demux/1 -> Trigonometric Function/1
  Selector3/1 -> Demux/1
  MATLAB Function/1(distance) -> d/1
  MATLAB Function/2(angle) -> Wrap to Pi1/1(In)
  Wrap to Pi1/1(Out) -> a/1

== system Follower_Agent/Data Models/Sensor Model1/Sense each vehicle/Radar Model2 ==
  Enable : EnablePort
  Bus Creator2 : BusCreator  Inputs=5  OutDataTypeStr=Bus: SensorData  NonVirtualBus=on
  Constant : Constant  Value=[100 0]
  Constant2 : Constant  Value=[ 0 0 0 ]
  Demux1 : Demux  Outputs=2
  Demux2 : Demux  Outputs=3
  Radar Data : Outport
  wires:
  Demux1/2 -> Bus Creator2/2  "azimuth"
  Demux1/1 -> Bus Creator2/1  "range"
  Demux2/3 -> Bus Creator2/5  "roadCurvature"
  Demux2/2 -> Bus Creator2/4  "headingError"
  Demux2/1 -> Bus Creator2/3  "lateralError"
  Bus Creator2/1 -> Radar Data/1
  Constant/1 -> Demux1/1
  Constant2/1 -> Demux2/1

== system Follower_Agent/Follower Vehicle Control/Platoon Steering Control1/Calculate lateral error1/Subsystem1 ==
  range : Inport
  azimuth : Inport  Port=2
  dPsi : Inport  Port=3
  MATLAB Function : MATLAB Function  TreatAsAtomicUnit=on
  Wrap to Pi2 : Subsystem
  distance : Outport
  angle : Outport  Port=2
  wires:
  dPsi/1 -> Wrap to Pi2/1(In)
  azimuth/1 -> MATLAB Function/2(theta_c)
  MATLAB Function/2(theta) -> angle/1
  Wrap to Pi2/1(Out) -> MATLAB Function/3(dpsi)
  MATLAB Function/1(d) -> distance/1
  range/1 -> MATLAB Function/1(d_r)

== system Follower_Agent/Follower Vehicle Control/Platoon Steering Control1/Calculate lateral error1/Wrap to Pi ==
  In : Inport
  Bias : Bias  Bias=pi
  Bias1 : Bias  Bias=-pi
  Constant : Constant  Value=2*pi
  Math Function : Math  Operator=mod  SaturateOnIntegerOverflow=on
  Out : Outport
  wires:
  In/1 -> Bias/1
  Bias/1 -> Math Function/1
  Math Function/1 -> Bias1/1
  Bias1/1 -> Out/1
  Constant/1 -> Math Function/2

== system Follower_Agent/Follower Vehicle Control/Variant Subsystem/Agent Control/Message Parser ==
  In1 : Inport
  Enable : EnablePort
  MATLAB Function : MATLAB Function  TreatAsAtomicUnit=on
  speed_control : Outport
  steering_control : Outport  Port=2
  spacing : Outport  Port=3
  wires:
  In1/1 -> MATLAB Function/1(buf)
  MATLAB Function/1(speed_control) -> speed_control/1
  MATLAB Function/2(steering_control) -> steering_control/1
  MATLAB Function/3(spacing) -> spacing/1

== system Follower_Agent/Follower Vehicle Control/Variant Subsystem/Agent Control/TCP Sockets ==
  Send : Inport
  function : TriggerPort  TriggerType=function-call
  Compare To Zero : simulink/Logic and Bit Operations/Compare To Zero  relop=>  OutDataTypeStr=boolean
  Constant : Constant  Value=zeros(16,1,'uint8')  OutDataTypeStr=uint8
  Level-2 MATLAB S-Function : M-S-Function  Priority=2  FunctionName=TCPReceive  Parameters='127.0.0.1',18000+vehicle-1,[16 1],1,0.5,-1,'uint8','LittleEndian'
  Level-2 MATLAB S-Function1 : M-S-Function  Priority=1  FunctionName=TCPSend  Parameters='127.0.0.1',17000+vehicle-1,0,0.5,'LittleEndian'
  Terminator : Terminator
  NewMessage : Outport
  Receive : Outport  Port=2
  wires:
  Level-2 MATLAB S-Function/1 -> Receive/1  "data"
  Send/1 -> Level-2 MATLAB S-Function1/1
  Level-2 MATLAB S-Function/2 -> Compare To Zero/1  "bytesReceived"
  Compare To Zero/1 -> NewMessage/1
  Constant/1 -> Level-2 MATLAB S-Function/1
  Level-2 MATLAB S-Function1/1 -> Terminator/1

== system Follower_Agent/Data Models/Sensor Model1/Sense each vehicle/Non-zero/Norm ==
  In1 : Inport
  Math Function : Math  Operator=square  SaturateOnIntegerOverflow=on
  Sqrt : Sqrt  SaturateOnIntegerOverflow=on
  Sum of Elements : Sum  Inputs=+
  Out1 : Outport
  wires:
  Math Function/1 -> Sum of Elements/1
  Sum of Elements/1 -> Sqrt/1
  Sqrt/1 -> Out1/1
  In1/1 -> Math Function/1
